simulink model "EKF_sim"  (R2020a)
settings: Solver=VariableStepAuto  StartTime=0.0  StopTime=694  RelTol=1e-3
values from neighbouring files (symbols this model uses):
  acc_variance = 4.8e-1    (= 0.48)    [init.m]
  bias_acc_variance = 4e-10    [init.m]
  bias_gyro_variance = 4e-14    [init.m]
  DT = EKF_DT    (= 0.02)    [init.m]
  EKF_DT = 0.02    [init.m]
  g = 9.81    [init.m]
  GPS_variance = 1e-2    (= 0.01)    [init.m]
  gyro_variance = 4.8e-2    (= 0.048)    [init.m]
  head_variance = 7e-3    (= 0.007)    [init.m]
  init_time = 11    [init.m]
  lambda_xa = 1e-4    (= 0.0001)    [init.m]
  lambda_xg = 1e-3    (= 0.001)    [init.m]
  SHOE_buffer_N = 100    [init.m]
  SHOE_threshold = 30    [init.m]
  t1_end = 291    [init.m]
  t1_start = 290    [init.m]
  t2_end = 392.5    [init.m]
  t2_start = 392    [init.m]
  t3_end = 420    [init.m]
  t3_start = 419    [init.m]
  t4_end = 439    [init.m]
  t4_start = 438    [init.m]
  vel_variance = 1e-2    (= 0.01)    [init.m]
  zero_vel_period = 50000    [init.m]
(part 5 of 5)

== matlab function EKF_sim/EKF_bias/System Update/virtual ==
  data: x_k input; R_ input; e output size=9 1; H output size=9 22; R_k output size=9 9; flag_updates_vector input; acc input; pos_GPS input; hea_GPS input; g parameter
% --------------------          virtual            -------------------- %
%{
% This function check the flag_updates_vector and produces the terms 'e',
% 'H' and 'R' based on it. When a flag update is set to zero by the
% previous function 'virtual', the dimensions of vector 'e' and matrices 
% 'H' and 'R' change to avoid wrong correction.
% There are three types of updates:

%  1. Zero Velocity constraints: we assume the vehicle moves only along its
%     x body axis direction, so the velocity in y and z axis are assumed to
%     be equal to zero.

%  2. No-accelerating mode: when we detect a very low acceleration of the
%     vehicle, we can assume the accelerometer measures the gravity vector.
%     In this case we can update roll and pitch angles.

%  3. Position and Yaw updates: when a new value from GPS is detected,
%     position and Yaw is updated.

% For more deatils about matrix 'H' and the change of dimension, see file
% 'calcolo_matrice_H' and 'cutter_matrix'.

% Input:
%     x_k                 : [22x1] state vector before correction step
%     R_                  : [9x9] Measurement Noise Covariance Matrix
%     flag_updates_vector : [3x1] flag vector for new updates
%     acc                 : [3x1] Accelerometer Measurement
%     pos_GPS             : [3x1] GPS data in NED
%     hea_GPS             : [1] Heading value from GPS data
%     g                   : gravity acceleration

% Output:
%     e         : [] Error between current measure and predicted measure
%     H         : [] Jacobian of prediction model measurement with respect  
%                 to state x
%     R_k       : [] Measurement Noise Covariance Matrix at time k
%}
%%
function [e, H, R_k] = virtual(x_k, R_, flag_updates_vector, acc, pos_GPS, hea_GPS, g)

    e = zeros(9,1);
    h = zeros(9,1);
    z = zeros(9,1);
    H = zeros(9,22);
    q = x_k(1:4);
    
    %Dynamical constraints update (zero velocity)
    if  flag_updates_vector(1) == 1
        %hv0 = zeros(3,1);
        v  = x_k(14:16);
        Rnb = fromq2rot(q(1),q(2),q(3),q(4));
        hv0 = Rnb'*v;
        
        %z = z + [0       0    0 0 0 0 0 0 0]';
        h = h + [hv0(2) hv0(3) 0 0 0 0 0 0 0]';
        
        [H(1,:), H(2,:)]= calcolo_Hv0(q(1),q(2),q(3),q(4),v(1),v(2),v(3));
    end
    
    %Roll and Pitch Updates    
    if flag_updates_vector(2) == 1
        %hg = zeros(3,1);
        Rnb = fromq2rot(q(1),q(2),q(3),q(4));
        hg = Rnb'*[0 0 -g]';
        
        xa = x_k(20:22);
        z = z + [0 0 acc(1)-xa(1) acc(2)-xa(2) acc(3)-xa(3) 0 0 0 0]';
        h = h + [0 0  hg(1)        hg(2)         hg(3)      0 0 0 0]';
        
        [H(3,:), H(4,:), H(5,:)]= calcolo_Hg(q(1),q(2),q(3),q(4),g);

    end
    
    %Position and Yaw Updates
    if flag_updates_vector(3) == 1
        
        r = x_k(11:13);
        % htheta = atan2(2*(q(2)*q(3)-q(1)*q(4)), 1-2*(q(3)^2+q(4)^2));
        var_yaw = atan2(2*(q(2)*q(3) + q(1)*q(4)), q(1)*q(1) + q(2)*q(2) - q(3)*q(3) - q(4)*q(4));
        
        z = z + [0 0 0 0 0 pos_GPS(1) pos_GPS(2) pos_GPS(3) hea_GPS]';
        h = h + [0 0 0 0 0    r(1)       r(2)       r(3)    var_yaw ]';
 
        H(6,:) = [0, 0, 0, 0, 0, 0, 0, 0, 0, 0, 1, 0, 0, 0, 0, 0, 0, 0, 0, 0, 0, 0];
        H(7,:) = [0, 0, 0, 0, 0, 0, 0, 0, 0, 0, 0, 1, 0, 0, 0, 0, 0, 0, 0, 0, 0, 0];
        H(8,:) = [0, 0, 0, 0, 0, 0, 0, 0, 0, 0, 0, 0, 1, 0, 0, 0, 0, 0, 0, 0, 0, 0];
        H(9,:)= calcolo_Htheta(q(1),q(2),q(3),q(4));  
    end
    e = z - h;
    coder.extrinsic('wrapToPi');
    if e(9)> pi
        e(9) = wrapToPi(e(9));
    end
    
    %After the generation of 'e', 'H' and 'R', we eliminate row and columns
    %of them if they are not used. The resultanting scaled vector and 
    %matrix are used in the next correction step function.
    R=R_;
    i=0;
    if  flag_updates_vector(1) == 0
        H(1-i,:) = [];
        e(1-i) = [];
        R(1-i,:) = [];
        R(:,1-i) = [];
        i=i+1;
        H(2-i,:) = [];
        e(2-i) = [];
        R(2-i,:) = [];
        R(:,2-i) = [];
        i=i+1;
    end
    if  flag_updates_vector(2) == 0
        H(3-i,:) = [];
        e(3-i) = [];
        R(3-i,:) = [];
        R(:,3-i) = [];
        i=i+1;
        H(4-i,:) = [];
        e(4-i) = [];
        R(4-i,:) = [];
        R(:,4-i) = [];
        i=i+1;
        H(5-i,:) = [];
        e(5-i) = [];
        R(5-i,:) = [];
        R(:,5-i) = [];
        i=i+1;
    end
    if  flag_updates_vector(3) == 0
        H(6-i,:) = [];
        e(6-i) = [];
        R(6-i,:) = [];
        R(:,6-i) = [];
        i=i+1;
        H(7-i,:) = [];
        e(7-i) = [];
        R(7-i,:) = [];
        R(:,7-i) = [];
        i=i+1;
        H(8-i,:) = [];
        e(8-i) = [];
        R(8-i,:) = [];
        R(:,8-i) = [];
        i=i+1;
        H(9-i,:) = [];
        e(9-i) = [];
        R(9-i,:) = [];
        R(:,9-i) = [];
    end
    R_k=R;
end

%% Auxiliary Functions
% This function computes the rotation matrix from quaternion
function rot = fromq2rot(q1,q2,q3,q4)
    rot = [q1^2+q2^2-q3^2-q4^2, 2*(q2*q3-q1*q4), 2*(q1*q3+q2*q4); ...
           2*(q2*q3+q1*q4), q1^2-q2^2+q3^2-q4^2, 2*(q3*q4-q1*q2); ...
           2*(q2*q4-q1*q3), 2*(q1*q2+q3*q4), q1^2-q2^2-q3^2+q4^2];
end
%%
% These functions calculate the H matrix elements
% See 'calcolo_matrice_H.m' for the symbolic calculation used
function [Hv01 , Hv02] = calcolo_Hv0(q1,q2,q3,q4,vx,vy,vz)  
    Hv01 = [ 2*q1*vy - 2*q4*vx + 2*q2*vz, 2*q3*vx - 2*q2*vy + 2*q1*vz, 2*q2*vx + 2*q3*vy + 2*q4*vz, 2*q3*vz - 2*q4*vy - 2*q1*vx, 0, 0, 0, 0, 0, 0, 0, 0, 0, 2*q2*q3 - 2*q1*q4, q1^2 - q2^2 + q3^2 - q4^2,2*q1*q2 + 2*q3*q4, 0, 0, 0, 0, 0, 0];
    Hv02 = [ 2*q3*vx - 2*q2*vy + 2*q1*vz, 2*q4*vx - 2*q1*vy - 2*q2*vz, 2*q1*vx + 2*q4*vy - 2*q3*vz, 2*q2*vx + 2*q3*vy + 2*q4*vz, 0, 0, 0, 0, 0, 0, 0, 0, 0, 2*q1*q3 + 2*q2*q4, 2*q3*q4 - 2*q1*q2, q1^2 - q2^2 - q3^2 + q4^2, 0, 0, 0, 0, 0, 0];
end
function [Hg1 , Hg2, Hg3] = calcolo_Hg(q1,q2,q3,q4,g)
    Hg1 = [  2*g*q3, -2*g*q4,  2*g*q1, -2*g*q2, 0, 0, 0, 0, 0, 0, 0, 0, 0, 0, 0, 0, 0, 0, 0, 0, 0, 0];
    Hg2 = [ -2*g*q2, -2*g*q1, -2*g*q4, -2*g*q3, 0, 0, 0, 0, 0, 0, 0, 0, 0, 0, 0, 0, 0, 0, 0, 0, 0, 0];
    Hg3 = [ -2*g*q1,  2*g*q2,  2*g*q3, -2*g*q4, 0, 0, 0, 0, 0, 0, 0, 0, 0, 0, 0, 0, 0, 0, 0, 0, 0, 0];
end
function Htheta= calcolo_Htheta(q1,q2,q3,q4)
    Htheta = [ (((2*q4)/(q1^2 + q2^2 - q3^2 - q4^2) - (2*q1*(2*q1*q4 + 2*q2*q3))/(q1^2 + q2^2 - q3^2 - q4^2)^2)*(q1^2 + q2^2 - q3^2 - q4^2)^2)/((2*q1*q4 + 2*q2*q3)^2 + (q1^2 + q2^2 - q3^2 - q4^2)^2), (((2*q3)/(q1^2 + q2^2 - q3^2 - q4^2) - (2*q2*(2*q1*q4 + 2*q2*q3))/(q1^2 + q2^2 - q3^2 - q4^2)^2)*(q1^2 + q2^2 - q3^2 - q4^2)^2)/((2*q1*q4 + 2*q2*q3)^2 + (q1^2 + q2^2 - q3^2 - q4^2)^2), (((2*q2)/(q1^2 + q2^2 - q3^2 - q4^2) + (2*q3*(2*q1*q4 + 2*q2*q3))/(q1^2 + q2^2 - q3^2 - q4^2)^2)*(q1^2 + q2^2 - q3^2 - q4^2)^2)/((2*q1*q4 + 2*q2*q3)^2 + (q1^2 + q2^2 - q3^2 - q4^2)^2), (((2*q1)/(q1^2 + q2^2 - q3^2 - q4^2) + (2*q4*(2*q1*q4 + 2*q2*q3))/(q1^2 + q2^2 - q3^2 - q4^2)^2)*(q1^2 + q2^2 - q3^2 - q4^2)^2)/((2*q1*q4 + 2*q2*q3)^2 + (q1^2 + q2^2 - q3^2 - q4^2)^2), 0, 0, 0, 0, 0, 0, 0, 0, 0,                 0,                         0,                         0, 0, 0, 0, 0, 0, 0];
end

%% %%%%%%%%%%%%%%%%%%%%%%%%%%%%%%%%%%%%%%%%%%%%%%%%%%%%%%%%%%%%%%%%%%%%%%%
     %%%%%%%%% Direct EKF for 6D Pose,  Marco Borraccino %%%%%%%%%%
     %%%%%%%%%   SGN Project, University of Pisa, 2021   %%%%%%%%%%
%%%%%%%%%%%%%%%%%%%%%%%%%%%%%%%%%%%%%%%%%%%%%%%%%%%%%%%%%%%%%%%%%%%%%%%%%%
